simulink model "PID_Controlled"  (R2018a)
settings: Solver=VariableStepAuto  StartTime=0.0  StopTime=10.0  RelTol=1e-3
libraries: simulink x1
settings Model: Creator=ABHISHEK  LastModifiedBy=ABHISHEK

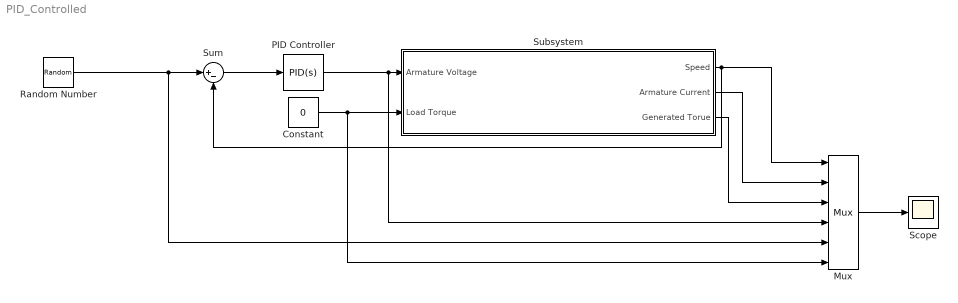
== system PID_Controlled ==
  Constant : Constant  Value=0
  Mux : Mux  Inputs=6
  PID Controller : simulink/Continuous/PID Controller  Controller=PID  TimeDomain=Continuous-time  SampleTime=-1  IntegratorMethod=Forward Euler  FilterMethod=Forward Euler  Form=Parallel  UseFilter=on  ControllerParametersSource=internal  P=0.07634  I=4.462  D=-0.006171  N=11.64  InitialConditionSource=internal  InitialConditionForIntegrator=0  InitialConditionForFilter=0  ExternalReset=none  LimitOutput=off  UpperSaturationLimit=inf  LowerSaturationLimit=-inf  LinearizeAsGain=on  AntiWindupMode=none  Kb=1  TrackingMode=off  Kt=1  PParamMin=[]  PParamMax=[]  IParamMin=[]  IParamMax=[]  DParamMin=[]  DParamMax=[]  NParamMin=[]  NParamMax=[]  KbParamMin=[]  KbParamMax=[]  KtParamMin=[]  KtParamMax=[]  POutMin=[]  POutMax=[]  IOutMin=[]  IOutMax=[]  DOutMin=[]  DOutMax=[]  NOutMin=[]  NOutMax=[]  KbOutMin=[]  KbOutMax=[]  KtOutMin=[]  KtOutMax=[]  IntegratorOutMin=[]  IntegratorOutMax=[]  FilterOutMin=[]  FilterOutMax=[]  SumOutMin=[]  SumOutMax=[]  SumI1OutMin=[]  SumI1OutMax=[]  SumI2OutMin=[]  SumI2OutMax=[]  SumI3OutMin=[]  SumI3OutMax=[]  SumDOutMin=[]  SumDOutMax=[]  SaturationOutMin=[]  SaturationOutMax=[]  IntegratorContinuousStateAttributes=''  IntegratorStateMustResolveToSignalObject=off  IntegratorRTWStateStorageClass=Auto  FilterContinuousStateAttributes=''  FilterStateMustResolveToSignalObject=off  FilterRTWStateStorageClass=Auto  DifferentiatorICPrevScaledInput=0  DifferentiatorOutMin=[]  DifferentiatorOutMax=[]  FilterDiffOutCoefMin=[]  FilterDiffOutCoefMax=[]  SumDenOutMin=[]  SumDenOutMax=[]  SumNumOutMin=[]  SumNumOutMax=[]  ReciprocalOutMin=[]  ReciprocalOutMax=[]  DivideOutMin=[]  DivideOutMax=[]  TunerSelectOption=Transfer Function Based (PID Tuner App)
  Random Number : RandomNumber  Mean=120  Variance=100  SampleTime=1
  Scope : Scope
  Subsystem : Subsystem
  Sum : Sum  Inputs=|+-
  wires:
  PID Controller/1 -> Mux/4, Subsystem/1("Armature Voltage ")
  Mux/1 -> Scope/1
  Subsystem/1("Speed ") -> Mux/1, Sum/2
  Subsystem/2(Armature Current) -> Mux/2
  Subsystem/3("Generated Torue ") -> Mux/3
  Random Number/1 -> Mux/5, Sum/1
  Constant/1 -> Subsystem/2("Load Torque "), Mux/6
  Sum/1 -> PID Controller/1

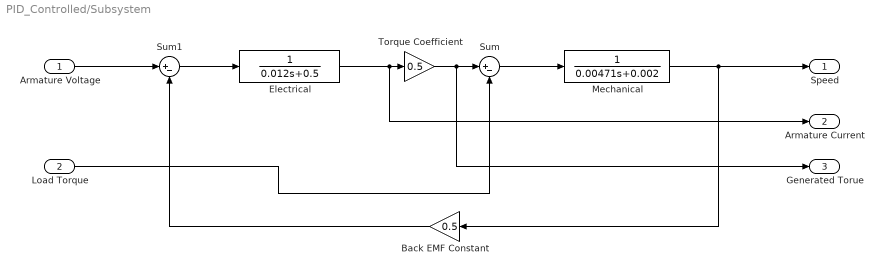
== system PID_Controlled/Subsystem ==
  "Armature Voltage " : Inport
  "Load Torque " : Inport  Port=2
  "Back EMF Constant " : Gain  Gain=0.5
  "Electrical " : TransferFcn  Denominator=[0.012 0.5]
  Mechanical : TransferFcn  Denominator=[0.00471 0.002]
  Sum : Sum  Inputs=|+-
  Sum1 : Sum  Inputs=|+-
  Torque Coefficient : Gain  Gain=0.5
  "Speed " : Outport
  Armature Current : Outport  Port=2
  "Generated Torue " : Outport  Port=3
  wires:
  "Back EMF Constant "/1 -> Sum1/2
  "Electrical "/1 -> Armature Current/1, Torque Coefficient/1
  Mechanical/1 -> "Speed "/1, "Back EMF Constant "/1
  "Armature Voltage "/1 -> Sum1/1
  Sum1/1 -> "Electrical "/1
  Torque Coefficient/1 -> "Generated Torue "/1, Sum/1
  Sum/1 -> Mechanical/1
  "Load Torque "/1 -> Sum/2
